simulink model "controller_sim"  (R2018a)
settings: Solver=VariableStepAuto  StartTime=0.0  StopTime=40.0  RelTol=1e-3
values from neighbouring files (symbols this model uses):
  A = import.A    [controller.m]    (also in response.m = [-1.48831293e-02 -1.70258267e-19  9.09646012e-01 -9.79307874; ss.mat = [-0.0156061059952 -0.102895241313 0.00225728292112 0 -0.0007)
  B = import.B    [controller.m]    (also in response.m = [0.00000000e+00  9.79307874e+00; ss.mat = [-0.571808844242  9.79282269132; -84.8106371027  1.740406975)
  C = double(import.C)    [controller.m]    (also in response.m = [1 0 0 0; ss.mat = [1 0 0 0 0 1 0 0 0 0 1 0 ... (16 elements, 4x4)])
  D = import.D    [controller.m]    (also in response.m = zeros(4,2); ss.mat = [0  0; 0  0; 0  0; 0  0])
  thetaf_initial = import.thetaf    [controller.m]
  u_initial = import.u    [controller.m]
  w_initial = import.w    [controller.m]
undefined symbols (not defined in the file or in its folder): sigbuilder_block
libraries: simulink_extras x4
settings Model: Creator=KILKISZenbook  LastModifiedBy=KILKISZenbook

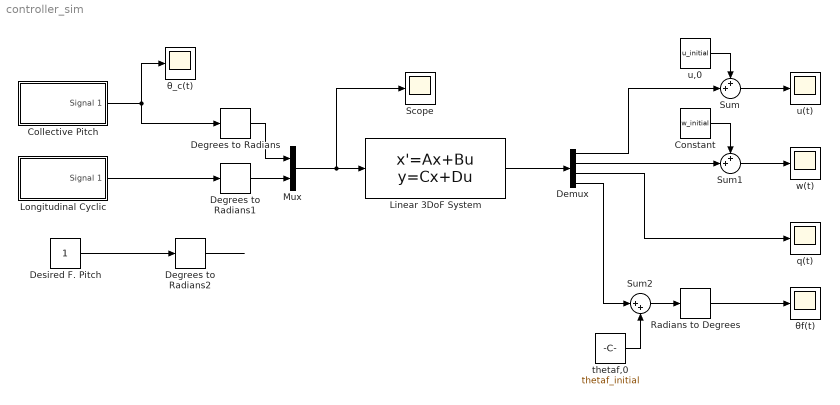
== system controller_sim ==
  Collective Pitch : Subsystem  Tag=STV Subsys  LoadFcn=sigbuilder_block('load');  StartFcn=sigbuilder_block('start');  StopFcn=sigbuilder_block('stop');  ClipboardFcn=sigbuilder_block('clipboard');  mask(Sigbuilder block){tuvar=[0:10]}
      mask help: Simulink:masks:SigbuilderBlock_MD
      mask init:
      | if ~strcmp(get_param(bdroot(gcbh),'SimulationStatus'),'stopped') tuvar = sigbuilder_block('maskInit'); end
      settings: CopyFcn=sigbuilder_block('copy');  DeleteFcn=sigbuilder_block('delete');  ModelCloseFcn=sigbuilder_block('modelClose');  PreSaveFcn=sigbuilder_block('preSave');  PauseFcn=sigbuilder_block('pause');  ContinueFcn=sigbuilder_block('continue');  NameChangeFcn=sigbuilder_block('namechange');  OpenFcn=sigbuilder_block('open',[437.6 199.2 550.4 400 ]);  CloseFcn=sigbuilder_block('close');
      mask Display: plot(0, 0, 100, 100,[2, 2, 32, 32, 2], [68, 8, 8, 68, 68],[32, 2], [38, 38], [32, 19, 2],[53, 60, 44], [32, 17, 17, 2],[16, 16, 31, 31]);txt = getActiveGroup(gcbh);text(2, 100, txt,'verticalAlignment', 'top');
  Constant : Constant  Value=w_initial
  Degrees to Radians : simulink_extras/Transformations/Degrees to Radians
  Degrees to Radians1 : simulink_extras/Transformations/Degrees to Radians
  Degrees to Radians2 : simulink_extras/Transformations/Degrees to Radians
  Demux : Demux
  Desired F. Pitch : Constant
  Linear 3DoF System : StateSpace  A=A  B=B  C=C  D=D  InitialCondition=0
  Longitudinal Cyclic : Subsystem  Tag=STV Subsys  LoadFcn=sigbuilder_block('load');  StartFcn=sigbuilder_block('start');  StopFcn=sigbuilder_block('stop');  ClipboardFcn=sigbuilder_block('clipboard');  mask(Sigbuilder block){tuvar=[0:10]}
      mask help: Simulink:masks:SigbuilderBlock_MD
      mask init:
      | if ~strcmp(get_param(bdroot(gcbh),'SimulationStatus'),'stopped') tuvar = sigbuilder_block('maskInit'); end
      settings: CopyFcn=sigbuilder_block('copy');  DeleteFcn=sigbuilder_block('delete');  ModelCloseFcn=sigbuilder_block('modelClose');  PreSaveFcn=sigbuilder_block('preSave');  PauseFcn=sigbuilder_block('pause');  ContinueFcn=sigbuilder_block('continue');  NameChangeFcn=sigbuilder_block('namechange');  OpenFcn=sigbuilder_block('open',[437.6 199.2 550.4 400 ]);  CloseFcn=sigbuilder_block('close');
      mask Display: plot(0, 0, 100, 100,[2, 2, 32, 32, 2], [68, 8, 8, 68, 68],[32, 2], [38, 38], [32, 19, 2],[53, 60, 44], [32, 17, 17, 2],[16, 16, 31, 31]);txt = getActiveGroup(gcbh);text(2, 100, txt,'verticalAlignment', 'top');
  Mux : Mux  Inputs=2
  Radians to Degrees : simulink_extras/Transformations/Radians to Degrees
  Scope : Scope
  Sum : Sum  Inputs=++|
  Sum1 : Sum  Inputs=++|
  Sum2 : Sum  Inputs=|++
  q(t) : Scope
  thetaf,0 : Constant  Value=thetaf_initial
  u(t) : Scope
  u,0 : Constant  Value=u_initial
  w(t) : Scope
  θ_c(t) : Scope
  θf(t) : Scope
  wires:
  Longitudinal Cyclic/1(Signal 1) -> Degrees to Radians1/1
  Demux/3 -> q(t)/1
  Linear 3DoF System/1 -> Demux/1
  Degrees to Radians/1 -> Mux/1
  Degrees to Radians1/1 -> Mux/2
  Collective Pitch/1(Signal 1) -> Degrees to Radians/1, θ_c(t)/1
  Sum/1 -> u(t)/1
  u,0/1 -> Sum/1
  Mux/1 -> Scope/1, Linear 3DoF System/1
  Constant/1 -> Sum1/1
  Demux/2 -> Sum1/2
  Sum1/1 -> w(t)/1
  Desired F. Pitch/1 -> Degrees to Radians2/1
  Degrees to Radians2/1 -> ?
  Demux/1 -> Sum/2
  Sum2/1 -> Radians to Degrees/1
  Demux/4 -> Sum2/1
  thetaf,0/1 -> Sum2/2
  Radians to Degrees/1 -> θf(t)/1

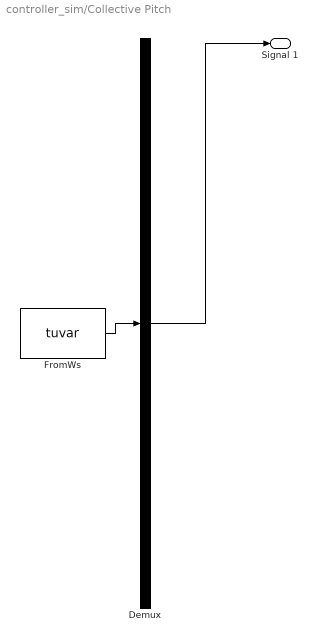
== system controller_sim/Collective Pitch ==
  Demux : Demux  Tag=STV Demux  Outputs=1
  FromWs : FromWorkspace  Tag=STV FromWs  VariableName=tuvar  SampleTime=0
      SigBuilderData=|
      | common.afterFinalStr = 'Extrapolate'
      | common.sampleTime = 0
      | dataSet.timeRange = [0 10]
      | dataSet.name = 'Group 1'
      | sbobj.Groups.Name = 'Group 1'
      | sbobj.Groups.Signals.Name = 'Signal 1'
      | sbobj.Groups.Signals.XData = [0 0.5 1 10]
      | sbobj.Groups.Signals.YData = [0 0 0 0]
  Signal 1 : Outport  Tag=STV Outport
  wires:
  Demux/1 -> Signal 1/1
  FromWs/1 -> Demux/1

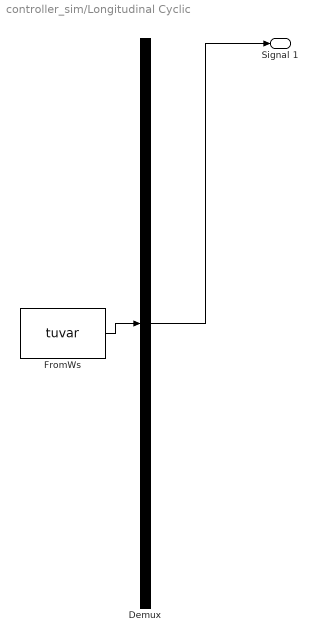
== system controller_sim/Longitudinal Cyclic ==
  Demux : Demux  Tag=STV Demux  Outputs=1
  FromWs : FromWorkspace  Tag=STV FromWs  VariableName=tuvar  SampleTime=0
      SigBuilderData=|
      | common.afterFinalStr = 'Extrapolate'
      | common.sampleTime = 0
      | dataSet.timeRange = [0 10]
      | dataSet.name = 'Group 1'
      | sbobj.Groups.Name = 'Group 1'
      | sbobj.Groups.Signals.Name = 'Signal 1'
      | sbobj.Groups.Signals.XData = [0 0.5 0.5 1 1 10]
      | sbobj.Groups.Signals.YData = [0 0 1 1 0 0]
  Signal 1 : Outport  Tag=STV Outport
  wires:
  Demux/1 -> Signal 1/1
  FromWs/1 -> Demux/1
